simulink model "sim_pert_sin"  (R2014b)
settings: Solver=ode45  StartTime=0.0  StopTime=10  MaxStep=0.001  RelTol=1e-3
values from neighbouring files (symbols this model uses):
  A = [0 -23.8095;0 0]    [Observador.m]    (also in P1.m; P1_pert.m; P1_pert_range.m; P1_pert_sin.m)
  B = [0;-23.8095]    [Observador.m]    (also in P1.m; P1_pert.m; P1_pert_range.m; P1_pert_sin.m)
  C = [1 0]    [Observador.m]    (also in P1.m; P1_pert.m = eye(2); P1_pert_range.m = eye(2); P1_pert_sin.m = eye(2))
  C_pert = eye(3)    [P1_pert.m]    (also in P1_pert_range.m = eye(5); P1_pert_sin.m = eye(4); P1_pert_sin_ct.m = eye(5); P1_pert_sin_ct_imag.m = eye(5))
  D = [0;0]    [Observador.m]    (also in P1.m; P1_pert.m; P1_pert_range.m; P1_pert_sin.m)
  gam_pert = [gam; 0]    [P1_pert.m]    (also in P1_pert_range.m = [gam; zeros(3,1)]; P1_pert_sin.m = [gam; 0; 0]; P1_pert_sin_ct.m = [gam; 0; 0; 0]; P1_pert_sin_ct_imag.m = [gam; 0; 0; 0])
  K_dis = acker(phi,gam,P_dis)    [Observador.m]    (also in P1.m; P1_pert.m; P1_pert_range.m; P1_pert_sin.m)
  L_pert = K_obs_dis_pert'    [P1_pert.m]    (also in P1_pert_range.m; P1_pert_sin.m; P1_pert_sin_ct.m; P1_pert_sin_ct_imag.m)
  phi_pert = [phi gam; 0 0 1]    [P1_pert.m]    (also in P1_pert_range.m = [phi gam*C_d [0;0]; zeros(2,2) phi_sin [0;0]; zeros(1,4) 1]; P1_pert_sin.m = [phi gam [0;0]; zeros(2) phi_sin]; P1_pert_sin_ct.m = [phi gam gam [0;0]; zeros(3,2) [1;0;0] [[0 0]; phi_sin]]; P1_pert_sin_ct_imag.m = [phi gam gam [0;0]; zeros(3,2) [1;0;0] [[0 0]; phi_sin]])
settings Model: Creator=student  LastModifiedBy=lluis
settings DataIOCC: SignalLoggingSaveFormat=ModelDataLogs
settings OptimizationCC: ExpressionDepthLimit=2147483647
settings DebuggingCC: UnderspecifiedInitializationDetection=Classic  MergeDetectMultiDrivingBlocksExec=none  FcnCallInpInsideContextMsg=EnableAllAsWarning  StateNameClashWarn=warning
settings GRTTargetCC: CombineOutputUpdateFcns=off  GRTInterface=on

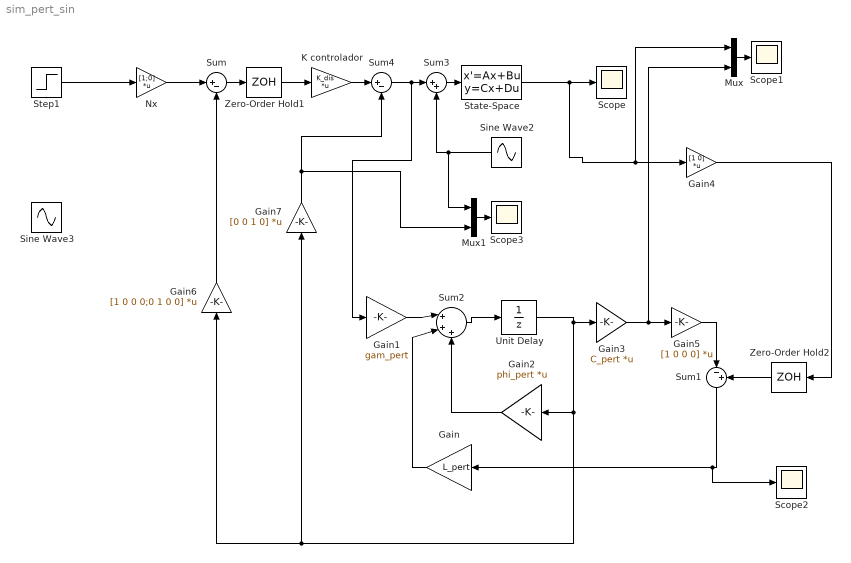
== system sim_pert_sin ==
  Gain : Gain  Gain=L_pert
  Gain1 : Gain  Gain=gam_pert
  Gain2 : Gain  Gain=phi_pert  Multiplication=Matrix(K*u)
  Gain3 : Gain  Gain=C_pert  Multiplication=Matrix(K*u)
  Gain4 : Gain  Gain=[1 0]  Multiplication=Matrix(K*u)
  Gain5 : Gain  Gain=[1 0 0 0]  Multiplication=Matrix(K*u)
  Gain6 : Gain  Gain=[1 0 0 0;0 1 0 0]  Multiplication=Matrix(K*u)
  Gain7 : Gain  Gain=[0 0 1 0]  Multiplication=Matrix(K*u)
  K controlador : Gain  Gain=K_dis  Multiplication=Matrix(K*u)
  Mux : Mux  Inputs=2
  Mux1 : Mux  Inputs=2
  Nx : Gain  Gain=[1;0]  Multiplication=Matrix(K*u)
  Scope{,1..3} (4 alike) : Scope
      Scope1 settings: TimeRange=10  YMin=-9.833064156845184e+215  YMax=8.962881488064375e+215
      Scope2 settings: SaveName=ScopeData2
      Scope3 settings: TimeRange=10  YMin=-9.833064156845184e+215  YMax=8.962881488064375e+215  SaveName=ScopeData3
  Sine Wave2 : Sin  Amplitude=0.1  Frequency=0.9319  SampleTime=0
  Sine Wave3 : Sin  Frequency=2  SampleTime=0
  State-Space : StateSpace  A=A  B=B  C=C  D=D  X0=[1;1]
  Step1 : Step  SampleTime=0
  Sum : Sum  Inputs=|+-
  Sum1 : Sum  Inputs=|-+
  Sum2 : Sum  Inputs=|+++
  Sum3 : Sum  Inputs=|++
  Sum4 : Sum  Inputs=|+-
  Unit Delay : UnitDelay  SampleTime=-1
  Zero-Order Hold1 : ZeroOrderHold  SampleTime=5E-2
  Zero-Order Hold2 : ZeroOrderHold  SampleTime=5E-2
  wires:
  State-Space/1 -> Mux/1, Gain4/1, Scope/1
  Sum/1 -> Zero-Order Hold1/1
  Step1/1 -> Nx/1
  Nx/1 -> Sum/1
  Zero-Order Hold1/1 -> K controlador/1
  Gain3/1 -> Mux/2, Gain5/1
  Sum1/1 -> Scope2/1, Gain/1
  Gain1/1 -> Sum2/1
  Gain/1 -> Sum2/2
  Unit Delay/1 -> Gain2/1, Gain7/1, Gain6/1, Gain3/1
  Sum2/1 -> Unit Delay/1
  Gain2/1 -> Sum2/3
  Gain4/1 -> Zero-Order Hold2/1
  Gain5/1 -> Sum1/1
  Mux/1 -> Scope1/1
  K controlador/1 -> Sum4/1
  Zero-Order Hold2/1 -> Sum1/2
  Sum3/1 -> State-Space/1
  Sine Wave2/1 -> Mux1/1, Sum3/2
  Gain6/1 -> Sum/2
  Sum4/1 -> Gain1/1, Sum3/1
  Gain7/1 -> Mux1/2, Sum4/2
  Mux1/1 -> Scope3/1
